simulink model "solucion"  (R2023a)
settings: Solver=FixedStepAuto  StartTime=0.0  StopTime=10.0  FixedStep=Ts  RelTol=1e-3
values from neighbouring files (symbols this model uses):
  refx = 5    [adjustTheta.m]
  refy = 1    [adjustTheta.m]
  Ts = 0.1    [adjustTheta.m]
settings Model: PacingRate=0.500000  Creator=jhon  LastModifiedBy=d.parras.2018

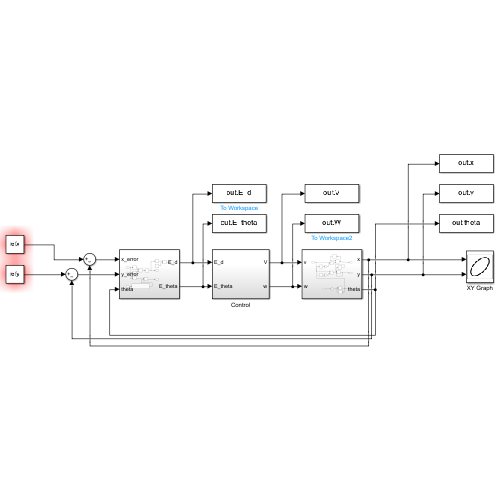
[thumbnail: Simulink's stored preview of the top-level diagram]
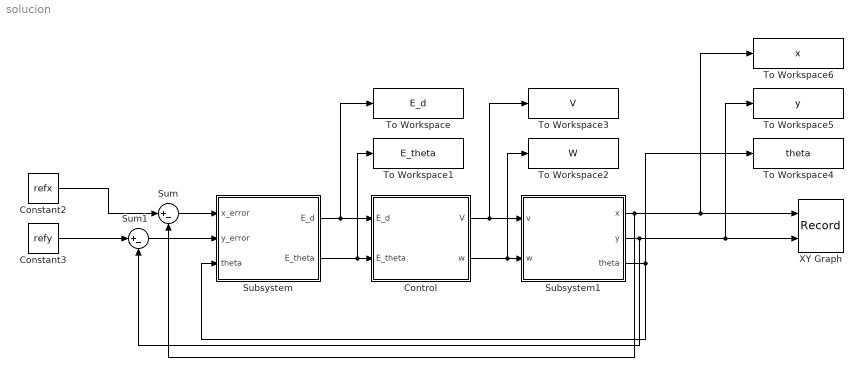
== system solucion ==
  Constant2 : Constant  Value=refx
  Constant3 : Constant  Value=refy
  Control : Subsystem
  Subsystem : Subsystem
  Subsystem1 : Subsystem
  Sum : Sum  Inputs=|+-
  Sum1 : Sum  Inputs=|+-
  To Workspace : ToWorkspace  VariableName=E_d  SaveFormat=Timeseries  SampleTime=-1
  To Workspace1 : ToWorkspace  VariableName=E_theta  SaveFormat=Timeseries  SampleTime=-1
  To Workspace2 : ToWorkspace  VariableName=W  SaveFormat=Timeseries  SampleTime=-1
  To Workspace3 : ToWorkspace  VariableName=V  SaveFormat=Timeseries  SampleTime=-1
  To Workspace4 : ToWorkspace  VariableName=theta  SaveFormat=Timeseries  SampleTime=-1
  To Workspace5 : ToWorkspace  VariableName=y  SaveFormat=Timeseries  SampleTime=-1
  To Workspace6 : ToWorkspace  VariableName=x  SaveFormat=Timeseries  SampleTime=-1
  XY Graph : Record  FileSettingsInternal="{\"entries\":[{\"content\":{\"excelSettings\":{\"content\":{},\"type\":\"Streamout.ExcelSettings\"}},\"type\":\"Streamout.FileSettingStorage\",\"uuid\":\"\"}],\"packageUris\":[\"http:\\/\\/schema.mathworks.com\\/mf0\\/streamout_blocks\\/R2020a\"],\"version\":\"1.0\"}"  Layout=[1 1]  SignalsInternal="{\"entries\":[{\"content\":{\"signals\":[{\"content\":{\"blockPath\":[],\"dimensions\":[1],\"domain\":\"\",\"lineColor\":\"#a2142f\",\"plots\":[1],\"port\":1,\"signalID\":1754,\"signalName\":\"XY Graph:1\"},\"type\":\"RecordBlkView.Signal\",\"uuid\":\"\"},{\"content\":{\"blockPath\":[],\"dimensions\":[1],\"domain\":\"\",\"lineColor\":\"#139fff\",\"plots\":[1],\"port\":2,\"signalID\":1757,\"signalName\":\"XY Graph:2\"},\"type\":\"RecordBlkView.Signal\",\"uuid\":\"\"}]},\"type\":\"RecordBlkView.InputSignals\",\"uuid\":\"\"}],\"packageUris\":[\"http:\\/\\/schema.mathworks.com\\/mf0\\/streamout_blocks\\/R2020a\"],\"version\":\"1.0\"}"  VisualizationBindings="{\"xyplotplugin\":{\"info\":[{\"series\":[{\"bindingParametersList\":[{\"parameter\":\"X-Axis\",\"signalID\":1754,\"signalName\":\"XY Graph:1\"},{\"parameter\":\"Y-Axis\",\"signalID\":1757,\"signalName\":\"XY Graph:2\"}],\"seriesID\":36590}],\"subplotID\":1}]}}"  CompatibilityTag=XY
  wires:
  Subsystem/1(E_d) -> To Workspace/1, Control/1(E_d)
  Subsystem/2(E_theta) -> To Workspace1/1, Control/2(E_theta)
  Control/1(V) -> To Workspace3/1, Subsystem1/1(v)
  Control/2(w) -> To Workspace2/1, Subsystem1/2(w)
  Subsystem1/1(x) -> Sum/2, To Workspace6/1, XY Graph/1
  Subsystem1/2(y) -> Sum1/2, To Workspace5/1, XY Graph/2
  Subsystem1/3(theta) -> Subsystem/3(theta), To Workspace4/1
  Sum/1 -> Subsystem/1(x_error)
  Sum1/1 -> Subsystem/2(y_error)
  Constant2/1 -> Sum/1
  Constant3/1 -> Sum1/1

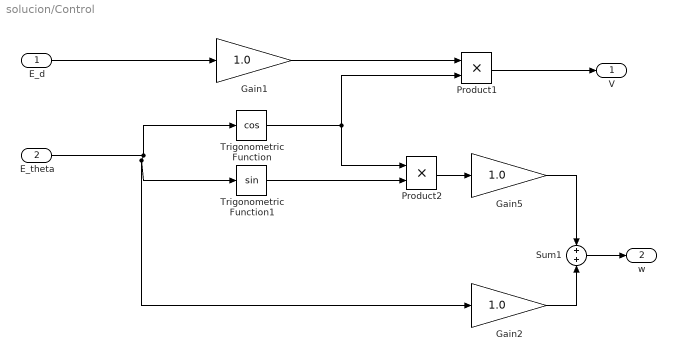
== system solucion/Control ==
  E_d : Inport
  E_theta : Inport  Port=2
  Gain1 : Gain  Gain=1.0
  Gain2 : Gain  Gain=1.0
  Gain5 : Gain  Gain=1.0
  Product1 : Product
  Product2 : Product
  Sum1 : Sum
  Trigonometric Function : Trigonometry  Operator=cos
  Trigonometric Function1 : Trigonometry
  V : Outport  VectorParamsAs1DForOutWhenUnconnected=off
  w : Outport  Port=2  VectorParamsAs1DForOutWhenUnconnected=off
  wires:
  E_theta/1 -> Trigonometric Function/1, Trigonometric Function1/1, Gain2/1
  E_d/1 -> Gain1/1
  Trigonometric Function/1 -> Product1/2, Product2/1
  Product1/1 -> V/1
  Trigonometric Function1/1 -> Product2/2
  Product2/1 -> Gain5/1
  Gain1/1 -> Product1/1
  Gain5/1 -> Sum1/1
  Gain2/1 -> Sum1/2
  Sum1/1 -> w/1

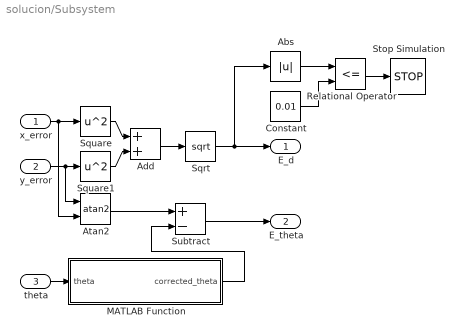
== system solucion/Subsystem ==
  x_error : Inport
  y_error : Inport  Port=2
  theta : Inport  Port=3
  Abs : Abs  SaturateOnIntegerOverflow=off
  Add : Sum
  Atan2 : Trigonometry  Operator=atan2
  Constant : Constant  Value=0.01
  MATLAB Function : MATLAB Function  TreatAsAtomicUnit=on
  Relational Operator : RelationalOperator  Operator=<=  OutDataTypeStr=boolean  RndMeth=Simplest  InputSameDT=off
  Sqrt : Sqrt
  Square : Math  Operator=square
  Square1 : Math  Operator=square
  Stop Simulation : Stop
  Subtract : Sum  Inputs=+-
  E_d : Outport
  E_theta : Outport  Port=2
  wires:
  x_error/1 -> Atan2/2, Square/1
  y_error/1 -> Atan2/1, Square1/1
  Square/1 -> Add/1
  Square1/1 -> Add/2
  Add/1 -> Sqrt/1
  Sqrt/1 -> Abs/1, E_d/1
  Atan2/1 -> Subtract/1
  Subtract/1 -> E_theta/1
  Constant/1 -> Relational Operator/2
  Abs/1 -> Relational Operator/1
  Relational Operator/1 -> Stop Simulation/1
  theta/1 -> MATLAB Function/1(theta)
  MATLAB Function/1(corrected_theta) -> Subtract/2

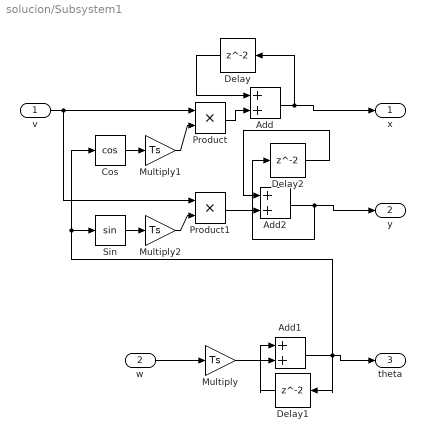
== system solucion/Subsystem1 ==
  v : Inport
  w : Inport  Port=2
  Add : Sum
  Add1 : Sum
  Add2 : Sum
  Cos : Trigonometry  Operator=cos
  Delay : Delay
  Delay1 : Delay
  Delay2 : Delay
  Multiply : Gain  Gain=Ts
  Multiply1 : Gain  Gain=Ts
  Multiply2 : Gain  Gain=Ts
  Product : Product
  Product1 : Product
  Sin : Trigonometry
  x : Outport
  y : Outport  Port=2
  theta : Outport  Port=3
  wires:
  w/1 -> Multiply/1
  Add/1 -> Delay/1, x/1
  Delay/1 -> Add/1
  Add1/1 -> Sin/1, Cos/1, Delay1/1, theta/1
  Multiply/1 -> Add1/2
  Delay1/1 -> Add1/1
  Cos/1 -> Multiply1/1
  Multiply1/1 -> Product/2
  v/1 -> Product1/1, Product/1
  Product/1 -> Add/2
  Sin/1 -> Multiply2/1
  Multiply2/1 -> Product1/2
  Product1/1 -> Add2/2
  Add2/1 -> Delay2/1, y/1
  Delay2/1 -> Add2/1

== matlab function solucion/Subsystem/MATLAB Function ==
  data: theta input; corrected_theta output
function corrected_theta = adjustTheta(theta)
    % Si theta es mayor o igual a pi, restarle 2*pi
    if theta >= pi
        corrected_theta = theta - 2*pi;
    % Si theta es menor o igual a -pi, sumarle 2*pi
    elseif theta <= -pi
        corrected_theta = theta + 2*pi;
    % En otros casos, no es necesario ajuste
    else
        corrected_theta = theta;
    end
end
